simulink model "bike"  (R2023b)
settings: Solver=VariableStepAuto  StartTime=0.0  StopTime=20  RelTol=1e-3
values from neighbouring files (symbols this model uses):
  C1 = 140*rad2deg    (= 8021.40913183)    [sim4.m]    (also in sim4_pt2.m = (C1r + C1l)*(180/pi))
  C2 = 140*rad2deg    (= 8021.40913183)    [sim4.m]    (also in sim4_pt2.m = (C2r + C2l)*(180/pi))
  Iz = 40000    [sim4.m]    (also in sim4_pt2.m = 1243.23988314)
  m = W / g    (= 93.2429912352)    [sim4.m]    (also in sim4_pt2.m)
  x1 = 3.5    [sim4.m]    (also in sim4_pt2.m)
  x2 = -4.5    [sim4.m]    (also in sim4_pt2.m)
settings Model: Creator=andres  LastModifiedBy=andres

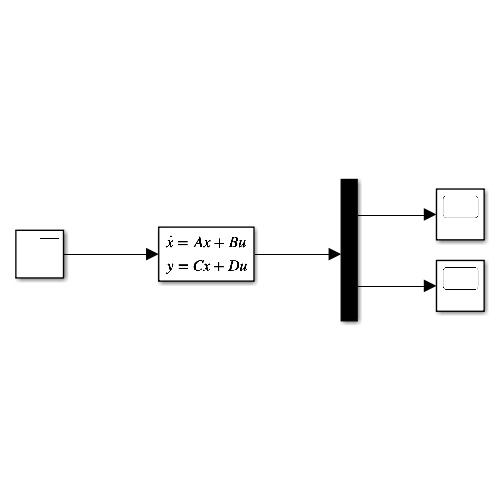
[thumbnail: Simulink's stored preview of the top-level diagram]
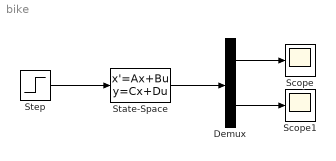
== system bike ==
  Demux : Demux  Outputs=2
  Scope : Scope
  Scope1 : Scope
  State-Space : StateSpace  A=[(-C1 - C2)/(m*u), ((-x1*x1*C1 - x2*x2*C2)/(m*u^2) - 1); (-x1*C1 - x2*C2)/(Iz), (-x1*x1*C1-x2*x2*C2)/(Iz*u)]  B=[C1/(m*u); x1*C1/Iz]  C=eye(2)  D=[0; 0]  InitialCondition=0
  Step : Step  After=0.02  SampleTime=0
  wires:
  Step/1 -> State-Space/1
  State-Space/1 -> Demux/1
  Demux/2 -> Scope1/1
  Demux/1 -> Scope/1
